simulink model "sprzezenie_od_stanu"  (R2017b)
settings: Solver=VariableStepAuto  StartTime=0.0  StopTime=10.0  RelTol=1e-3
values from neighbouring files (symbols this model uses):
  A2 = A1'    [initial_values.m]    (also in matlab.mat = [3.22791678547  1  0; -1.44925930399  0  1; 0.17377394345  0)
  B2 = C1'    [initial_values.m]    (also in matlab.mat = [0.260707487539 -0.289205764977 0.0761198486843])
  K = [-150 -150 -150]    [matlab.mat]    (also in pkt10.m = acker(A2,B2,[0.25,0.2+0.1i,-0.1i]); pkt6rzeczywiste.m = acker(A2,B2,[pole,pole,pole]); pkt6zespolone.m = acker(A2,B2,[zb1,zb2,zb3]); pkt7.m = Kpol(iter,:))
  Tp = 0.25    [initial_values.m]    (also in matlab.mat)
  X0 = [8 2 -1]    [pkt10.m]    (also in pkt6rzeczywiste.m; pkt6zespolone.m; pkt7.m; pkt7best.m)
settings Model: Creator=Paweł  LastModifiedBy=Paweł

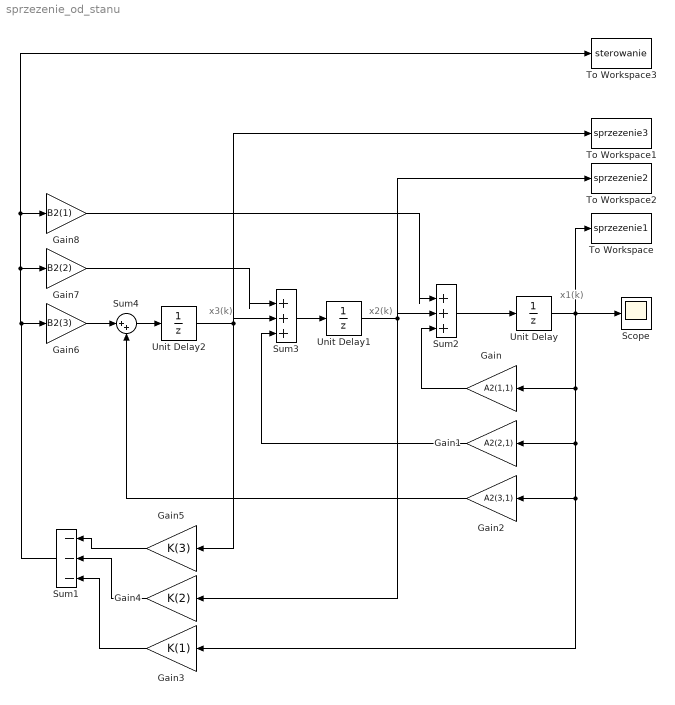
== system sprzezenie_od_stanu ==
  note: x1(k)
  note: x3(k)
  note: x2(k)
  Gain : Gain  Gain=A2(1,1)
  Gain1 : Gain  Gain=A2(2,1)
  Gain2 : Gain  Gain=A2(3,1)
  Gain3 : Gain  Gain=K(1)
  Gain4 : Gain  Gain=K(2)
  Gain5 : Gain  Gain=K(3)
  Gain6 : Gain  Gain=B2(3)
  Gain7 : Gain  Gain=B2(2)
  Gain8 : Gain  Gain=B2(1)
  Scope : Scope
  Sum1 : Sum  Inputs=---
  Sum2 : Sum  Inputs=|+++
  Sum3 : Sum  Inputs=|+++
  Sum4 : Sum  Inputs=|++
  To Workspace : ToWorkspace  VariableName=sprzezenie1  SaveFormat=Timeseries  SampleTime=-1
  To Workspace1 : ToWorkspace  VariableName=sprzezenie3  SaveFormat=Timeseries  SampleTime=-1
  To Workspace2 : ToWorkspace  VariableName=sprzezenie2  SaveFormat=Timeseries  SampleTime=-1
  To Workspace3 : ToWorkspace  VariableName=sterowanie  SaveFormat=Timeseries  SampleTime=-1
  Unit Delay : UnitDelay  InitialCondition=X0(1)  SampleTime=Tp
  Unit Delay1 : UnitDelay  InitialCondition=X0(2)  SampleTime=Tp
  Unit Delay2 : UnitDelay  InitialCondition=X0(3)  SampleTime=Tp
  wires:
  Sum1/1 -> To Workspace3/1, Gain8/1, Gain7/1, Gain6/1
  Gain2/1 -> Sum4/2
  Gain1/1 -> Sum3/3
  Gain5/1 -> Sum1/1
  Gain4/1 -> Sum1/2
  Gain3/1 -> Sum1/3
  Unit Delay1/1 -> To Workspace2/1, Gain4/1, Sum2/2
  Gain/1 -> Sum2/3
  Sum4/1 -> Unit Delay2/1
  Gain7/1 -> Sum3/1
  Unit Delay/1 -> Gain3/1, Gain2/1, Gain1/1, Gain/1, Scope/1, To Workspace/1
  Sum3/1 -> Unit Delay1/1
  Unit Delay2/1 -> To Workspace1/1, Gain5/1, Sum3/2
  Gain6/1 -> Sum4/1
  Sum2/1 -> Unit Delay/1
  Gain8/1 -> Sum2/1
